simulink model "bondarko3Task"  (R2013a)
settings: Solver=ode45  SolverMode=SingleTasking  StartTime=0.0  StopTime=10.0  RelTol=1e-3
undefined symbols (not defined in the file): K, T
settings Model: CovMetricSettings=dwe  CovHtmlReporting=off  covSaveCumulativeToWorkspaceVar=off  CovSaveSingleToWorkspaceVar=off  CovExternalEMLEnable=on  Creator=Петр  LastModifiedBy=Петр
settings DataIOCC: LimitDataPoints=off  SaveFormat=StructureWithTime
settings DebuggingCC: UnderspecifiedInitializationDetection=Simplified  MergeDetectMultiDrivingBlocksExec=error  SolverPrmCheckMsg=none  FrameProcessingCompatibilityMsg=error  StateNameClashWarn=none  SFUnexpectedBacktrackingDiag=error  SFNoUnconditionalDefaultTransitionDiag=error
settings HardwareCC: ProdBitPerPointer=64  ProdLargestAtomicFloat=Float  ProdIntDivRoundTo=Zero  ProdEndianess=LittleEndian  ProdHWDeviceType=Specified
settings ModelReferenceCC: PropagateSignalLabelsOutOfModel=on
settings GRTTargetCC: CodeReplacementLibrary=C99 (ISO)  GeneratePreprocessorConditionals=Use local settings

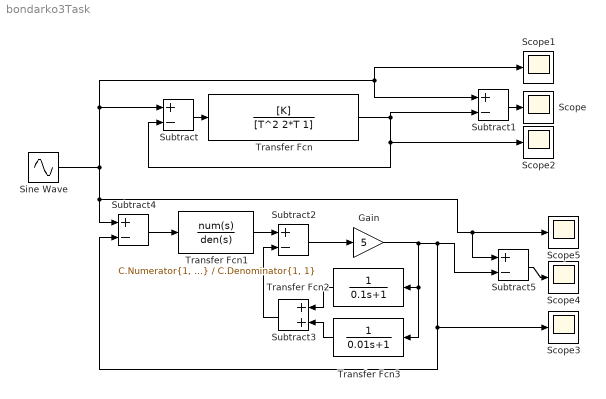
== system bondarko3Task ==
  Gain : Gain  Gain=5
  Scope{,1..5} (6 alike) : Scope
      Scope settings: TimeRange=auto  MaxDataPoints=5000  SaveToWorkspace=off  SaveName=ScopeData  YMin=-0.02543  YMax=0.02542  SampleTime=-1
      Scope1 settings: TimeRange=auto  MaxDataPoints=5000  SaveToWorkspace=off  YMin=-1.25  YMax=1.25  SampleTime=-1
      Scope2 settings: TimeRange=auto  MaxDataPoints=5000  SaveToWorkspace=off  SaveName=ScopeData2  YMin=-1.22536  YMax=1.22537  SampleTime=-1
      Scope3 settings: TimeRange=auto  MaxDataPoints=5000  SaveToWorkspace=off  YMin=-1.2253  YMax=1.22554  SampleTime=-1
      Scope4 settings: TimeRange=auto  MaxDataPoints=5000  SaveToWorkspace=off  SaveName=ScopeData2  YMin=-0.02592  YMax=0.02538  SampleTime=-1
      Scope5 settings: TimeRange=auto  MaxDataPoints=5000  SaveToWorkspace=off  SaveName=ScopeData3  YMin=-1.25  YMax=1.25  SampleTime=-1
  Sine Wave : Sin  Frequency=2*pi  SampleTime=0
  Subtract{,1..2,4..5} (5 alike) : Sum  Inputs=+-
  Subtract3 : Sum
  Transfer Fcn : TransferFcn  Numerator=[K]  Denominator=[T^2 2*T 1]
  Transfer Fcn1 : TransferFcn  Numerator=C.Numerator{1, 1}  Denominator=C.Denominator{1, 1}
  Transfer Fcn2 : TransferFcn  Denominator=[0.1 1]
  Transfer Fcn3 : TransferFcn  Denominator=[0.01 1]
  wires:
  Subtract/1 -> Transfer Fcn/1
  Transfer Fcn/1 -> Subtract1/2, Subtract/2, Scope2/1
  Subtract1/1 -> Scope/1
  Sine Wave/1 -> Scope1/1, Subtract1/1, Subtract/1, Scope5/1, Subtract5/1, Subtract4/1
  Transfer Fcn1/1 -> Subtract2/1
  Subtract2/1 -> Gain/1
  Transfer Fcn2/1 -> Subtract3/1
  Transfer Fcn3/1 -> Subtract3/2
  Subtract3/1 -> Subtract2/2
  Subtract4/1 -> Transfer Fcn1/1
  Subtract5/1 -> Scope4/1
  Gain/1 -> Subtract5/2, Subtract4/2, Scope3/1, Transfer Fcn3/1, Transfer Fcn2/1
